simulink model "AproximateModel"  (R2019b)
settings: Solver=FixedStepDiscrete  StartTime=0.0  StopTime=1  RelTol=1e-3
settings Model: Creator=Алексей  LastModifiedBy=Алексей
settings RTWCC: GenCodeOnly=on  PackageGeneratedCodeAndArtifacts=on

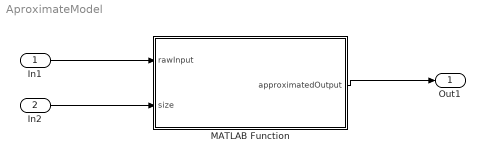
== system AproximateModel ==
  In1 : Inport  OutDataTypeStr=fixdt(1,16,2^0,0)  LockScale=on
  In2 : Inport  Port=2  OutDataTypeStr=int16
  MATLAB Function : MATLAB Function  TreatAsAtomicUnit=on
  Out1 : Outport  OutDataTypeStr=fixdt(1,16,2^0,0)
  wires:
  In1/1 -> MATLAB Function/1(rawInput)
  MATLAB Function/1(approximatedOutput) -> Out1/1
  In2/1 -> MATLAB Function/2(size)

== matlab function AproximateModel/MATLAB Function ==
  data: rawInput input; size input; approximatedOutput output
function approximatedOutput = fcn(rawInput, size)
Input = rawInput(1:size);
x = 1:1:length(Input);
x = rot90(x);
coeff2 = polyfit(x, Input, 5);
approximatedOutput = coeff2;
